simulink model "Trans_2016_DIF_M2_bez_oscilograf"  (R2015a)
settings: Solver=ode23tb  StartTime=0.0  StopTime=4  FixedStep=4e-6  MaxStep=1e-5  RelTol=1e-3  AbsTol=1e-5
values from neighbouring files (symbols this model uses):
  f = 50    [matlab.mat]
  Gm = 6.28318530718e-07    [matlab.mat]
  k = k+1    (= 2)    [SIGMA_trans.m]    (also in matlab.mat = 1e-06)
  LL1 = 0.016    [matlab.mat]
  LL2 = 7.96e-06    [matlab.mat]
  Ln = 0.0060919505207    [matlab.mat]
  R1 = 3.03    [matlab.mat]
  R2 = 0.003    [matlab.mat]
  RL1 = 10    [matlab.mat]
  RL2 = 0.00125    [matlab.mat]
  Rn = 0.63798571162    [matlab.mat]
  S = 0.0216    [matlab.mat]
  w1 = 850    [matlab.mat]
  w2 = 34    [matlab.mat]
undefined symbols (not defined in the file): Lsigma, sigma1, sigma2
libraries: powerlib x77, simulink x1
(part 1 of 2)
settings Model: Creator=Алексей  LastModifiedBy=Aleksey
settings SolverCC: MaxOrder=2  MaxConsecutiveZCs=5.5e6  NumberNewtonIterations=10000  MaxConsecutiveMinStep=1e7  ShapePreserveControl=EnableAll  ZeroCrossAlgorithm=Adaptive  SolverResetMethod=Robust  InsertRTBMode=Always

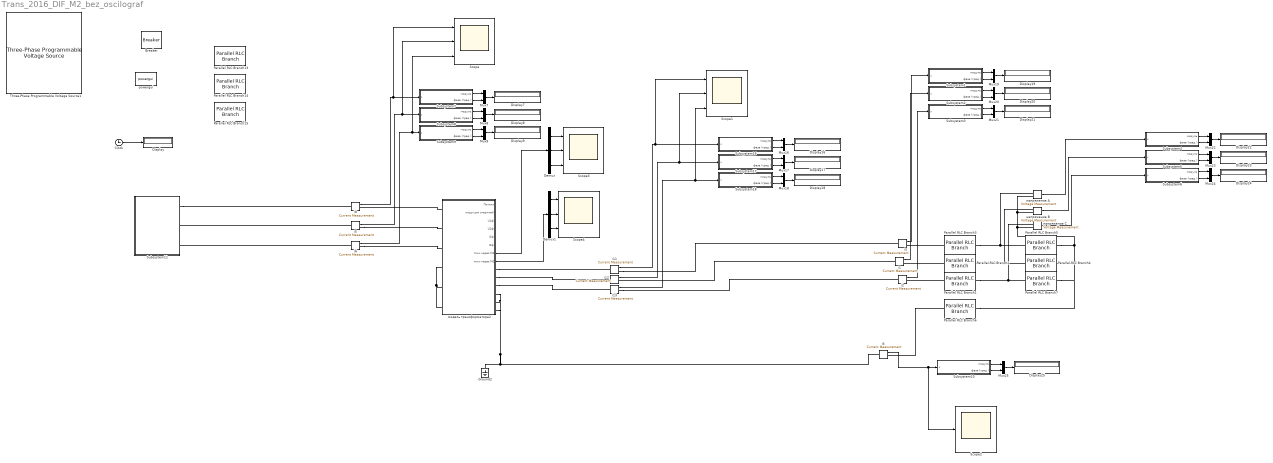
== system Trans_2016_DIF_M2_bez_oscilograf ==
  Breaker : powerlib/Elements/Breaker  InitialState=0  SwitchingTimes="[0.5  2]"  External=off  BreakerResistance=0.01  SnubberResistance=1e6  SnubberCapacitance=inf  Measurements=None  MoreParameters=on  NoBreakLoop=off
  Clock : Clock
  Demux : Demux  Outputs=3
  Demux1 : Demux  Outputs=3
  Display{,7..9,16..25} (14 alike) : Display
      Display16 settings: Decimation=2
      Display17 settings: Decimation=2
      Display18 settings: Decimation=2
      Display19 settings: Decimation=2
      Display20 settings: Decimation=2
      Display21 settings: Decimation=2
      Display22 settings: Decimation=2
      Display23 settings: Decimation=2
      Display24 settings: Decimation=2
      Display25 settings: Decimation=2
      Display7 settings: Decimation=2
      Display8 settings: Decimation=2
      Display9 settings: Decimation=2
  Ground2 : powerlib/Elements/Ground  LConnTagsString=a
  Mux{7..9,16..25} (13 alike) : Mux  Inputs=2
  Parallel RLC Branch{1..3,6} (4 alike) : powerlib/Elements/Parallel RLC Branch  LConnTagsString=a  RConnTagsString=__new0  BranchType=RL  Resistance=RL2  Inductance=LL2  SetiL0=off  InitialCurrent=0  Capacitance=1e-6  Setx0=off  InitialVoltage=0  Measurements=None
  Parallel RLC Branch13 : powerlib/Elements/Parallel RLC Branch  LConnTagsString=a  RConnTagsString=__new0  BranchType=RL  Resistance=RL1  Inductance=LL1  SetiL0=off  InitialCurrent=0  Capacitance=1e-6  Setx0=off  InitialVoltage=0  Measurements=None
  Parallel RLC Branch14 : powerlib/Elements/Parallel RLC Branch  LConnTagsString=a  RConnTagsString=__new0  BranchType=RL  Resistance=RL1  Inductance=LL1  SetiL0=off  InitialCurrent=0  Capacitance=1e-6  Setx0=off  InitialVoltage=0  Measurements=None
  Parallel RLC Branch15 : powerlib/Elements/Parallel RLC Branch  LConnTagsString=a  RConnTagsString=__new0  BranchType=RL  Resistance=RL1  Inductance=LL1  SetiL0=off  InitialCurrent=0  Capacitance=1e-6  Setx0=off  InitialVoltage=0  Measurements=None
  Parallel RLC Branch4 : powerlib/Elements/Parallel RLC Branch  LConnTagsString=a  RConnTagsString=__new0  BranchType=RL  Resistance=Rn  Inductance=Ln  SetiL0=off  InitialCurrent=0  Capacitance=1e-6  Setx0=off  InitialVoltage=0  Measurements=None
  Parallel RLC Branch5 : powerlib/Elements/Parallel RLC Branch  LConnTagsString=a  RConnTagsString=__new0  BranchType=RL  Resistance=Rn  Inductance=Ln  SetiL0=off  InitialCurrent=0  Capacitance=1e-6  Setx0=off  InitialVoltage=0  Measurements=None
  Parallel RLC Branch7 : powerlib/Elements/Parallel RLC Branch  LConnTagsString=a  RConnTagsString=__new0  BranchType=RL  Resistance=Rn  Inductance=Ln  SetiL0=off  InitialCurrent=0  Capacitance=1e-6  Setx0=off  InitialVoltage=0  Measurements=None
  Scope{,1,3..4} (4 alike) : Scope  NumInputPorts=3
      Scope settings: YMin=-19.75~-3.5~15  YMax=-16~5~19.25  MaxDataPoints=20
      Scope1 settings: YMin=-550~-550~-550  YMax=550~550~550  MaxDataPoints=20
      Scope3 settings: YMin=-4~-1~-7.5e-126  YMax=-2.4~1~1.25e-125  SaveName=ScopeData3  MaxDataPoints=20
      Scope4 settings: YMin=2.5e-11~-5.25e-10~1.35e-10  YMax=4e-10~-2.25e-10~2.15e-10  SaveName=ScopeData4  MaxDataPoints=20
  Scope2 : Scope
      settings: YMin=-1  YMax=0.4  SaveName=ScopeData2  MaxDataPoints=20
  Subsystem1 : Subsystem  mask{f=f}
      mask prompts: f "частота"
  Subsystem10 : Subsystem  mask{f=f}
      mask prompts: f "частота"
  Subsystem11 : Subsystem  mask{U=10000, Usek=10000*10/2, f=50}
      mask prompts: U "Линейное U"; Usek "на сколько вырастет напряжение за с"; f "частота"
      mask DialogControl ParameterGroupVar Prompt: Параметры
  Subsystem16 : Subsystem  mask{f=f}
      mask prompts: f "частота"
  Subsystem17 : Subsystem  mask{f=f}
      mask prompts: f "частота"
  Subsystem18 : Subsystem  mask{f=f}
      mask prompts: f "частота"
  Subsystem2 : Subsystem  mask{f=f}
      mask prompts: f "частота"
  Subsystem3 : Subsystem  mask{f=f}
      mask prompts: f "частота"
  Subsystem4 : Subsystem  mask{f=f}
      mask prompts: f "частота"
  Subsystem5 : Subsystem  mask{f=f}
      mask prompts: f "частота"
  Subsystem6 : Subsystem  mask{f=f}
      mask prompts: f "частота"
  Subsystem7 : Subsystem  mask{f=f}
      mask prompts: f "частота"
  Subsystem8 : Subsystem  mask{f=f}
      mask prompts: f "частота"
  Subsystem9 : Subsystem  mask{f=f}
      mask prompts: f "частота"
  Three-Phase Programmable Voltage Source1 : powerlib/Electrical Sources/Three-Phase Programmable Voltage Source  PositiveSequence="[0.01  50 50]"  VariationEntity=Amplitude  VariationType=Ramp  VariationTypeAlt=Step  VariationStep=0.5  VariationRate=10000/sqrt(3)*100*1.225/0.2  VariationMagnitude=0.3  VariationFrequency=2  VariationTiming=[0 0.2]  VariationPhaseA=off  Amplitudes=[1 0.8 1.2 1.0]  TimeValues=[0 0.1 0.15 0.2]  HarmonicGeneration=off  HarmonicA=[3 0.2 -25 0]  HarmonicB=[2 0.15 35 2]  Timing="[0.05  3]"  BusType=swing  Pref=0  Qref=0  Qmin=-inf  Qmax=inf
  i{1..6,8,11..13} (10 alike) : powerlib/Measurements/Current Measurement  PhasorSimulation=off  OutputType=Complex  PSBequivalent=0
  powergui : powerlib/powergui  Priority=1  SimulationMode=Continuous  SolverType=Tustin/Backward Euler (TBE)  SampleTime=50e-6  frequency=60  SPID=off  DisableSnubberDevices=off  DisableRonSwitches=off  DisableVfSwitches=off  SwTol=0  DisplayEquations=off  Interpol=off  methode=off  Ts=100  FunctionMessages=off  echomessages=off  HookPort=off  EnableUseOfTLC=off  x0status=blocks  frequencyindice=0  Pbase=100e6  ErrMax=1e-4  Iterations=50  UnitsV=kV  UnitsW=MW  buscounter=0  RestoreLinks=warning  ResistiveCurrentMeasurement=off  Frange=[0:2:500]  Ylog=off  Xlog=on  ShowGrid=off  save=off  variable=ZData  structure=0  ZoomFFT=off  StartTime=0.0  cycles=1  DisplayStyle=1  fundamental=60  FreqAxis=off  MaxFrequency=1000  frequencyindicesteady=1  RmsSteady=1  display=off
  модель трансформатора2 : Subsystem  mask{S=S, w1=w1, w2=w2, R1=R1, R2=R2, Lsigmavx=Lsigma, Sigma1=sigma1, Sigma2=sigma2, Gm=Gm, w1_do=[850 850 850], w2_do=[34 34 34], w1_posle=[850-21 850-21 850-21], w2_posle=[34 34 34], tRPN=0.3, tstup=0.1}
      mask prompts: S "Площадь сердечника"; w1 "Номинальное количество витков в первичной обмотке"; w2 "Номинальное количество витков в вторичной обмотке"; R1 "Активное сопротивление проводов первичной обмотки"; R2 "Сопротивление проводов вторичной обмотки"; Lsigmavx "индуктивность расеивания обмоток (квадратная матрица)"; Sigma1 "Участок сигма 1"; Sigma2 "Участок сигма 2"; Gm "Проводимость по воздуху"; w1_do "Матрица витков в первичке до срабатывания (1x3)"; w2_do "Матрица витков во вторичке до срабатывания (1x3)"; w1_posle "Матрица витков в первичке после срабатывания (1x3)"; w2_posle "Матрица витков во вторичке после срабатывания (1x3)"; tRPN "Время срабаотывания РПН"; tstup "Время шага ступени"
      mask DialogControl Container3 Prompt: Кривая намагничивания (матрицы должы быть одной размерности)
  напряжение А : powerlib/Measurements/Voltage Measurement  PhasorSimulation=off  OutputType=Complex  PSBequivalent=0
  напряжение В : powerlib/Measurements/Voltage Measurement  PhasorSimulation=off  OutputType=Complex  PSBequivalent=0
  напряжение С : powerlib/Measurements/Voltage Measurement  PhasorSimulation=off  OutputType=Complex  PSBequivalent=0
  wires:
  Clock/1 -> Display/1
  i3/1 -> Subsystem1/1(х)
  i1/1 -> Subsystem2/1(х)
  i2/1 -> Subsystem3/1(х)
  напряжение С/1 -> Subsystem6/1(х)
  напряжение В/1 -> Subsystem5/1(х)
  напряжение А/1 -> Subsystem4/1(х)
  i13/1 -> Scope1/3, Subsystem18/1(х)
  i11/1 -> Scope1/1, Subsystem16/1(х)
  Subsystem7/1(модуль) -> Mux7/1
  Subsystem7/2(фаза (град.)) -> Mux7/2
  Mux7/1 -> Display7/1
  Subsystem8/1(модуль) -> Mux8/1
  Subsystem8/2(фаза (град.)) -> Mux8/2
  Mux8/1 -> Display8/1
  Subsystem9/1(модуль) -> Mux9/1
  Subsystem9/2(фаза (град.)) -> Mux9/2
  Mux9/1 -> Display9/1
  Subsystem16/1(модуль) -> Mux16/1
  Subsystem16/2(фаза (град.)) -> Mux16/2
  Mux16/1 -> Display16/1
  Subsystem17/1(модуль) -> Mux17/1
  Subsystem17/2(фаза (град.)) -> Mux17/2
  Mux17/1 -> Display17/1
  Subsystem18/1(модуль) -> Mux18/1
  Subsystem18/2(фаза (град.)) -> Mux18/2
  Mux18/1 -> Display18/1
  Subsystem1/1(модуль) -> Mux19/1
  Subsystem1/2(фаза (град.)) -> Mux19/2
  Mux19/1 -> Display19/1
  Subsystem2/1(модуль) -> Mux20/1
  Subsystem2/2(фаза (град.)) -> Mux20/2
  Mux20/1 -> Display20/1
  Subsystem3/1(модуль) -> Mux21/1
  Subsystem3/2(фаза (град.)) -> Mux21/2
  Mux21/1 -> Display21/1
  Subsystem4/1(модуль) -> Mux22/1
  Subsystem4/2(фаза (град.)) -> Mux22/2
  Mux22/1 -> Display22/1
  Subsystem5/1(модуль) -> Mux23/1
  Subsystem5/2(фаза (град.)) -> Mux23/2
  Mux23/1 -> Display23/1
  Subsystem6/1(модуль) -> Mux24/1
  Subsystem6/2(фаза (град.)) -> Mux24/2
  Mux24/1 -> Display24/1
  Subsystem10/2(фаза (град.)) -> Mux25/2
  Mux25/1 -> Display25/1
  Subsystem10/1(модуль) -> Mux25/1
  i8/1 -> Scope/1, Subsystem7/1(х)
  i5/1 -> Subsystem8/1(х), Scope/2
  i6/1 -> Scope/3, Subsystem9/1(х)
  i12/1 -> Scope1/2, Subsystem17/1(х)
  i4/1 -> Scope2/1, Subsystem10/1(х)
  Demux/1 -> Scope3/1
  Demux/2 -> Scope3/2
  Demux/3 -> Scope3/3
  модель трансформатора2/7(токи через М1) -> Demux/1
  Demux1/1 -> Scope4/1
  Demux1/2 -> Scope4/2
  Demux1/3 -> Scope4/3
  модель трансформатора2/8(токи через М2) -> Demux1/1
  connections:
  модель трансформатора2/RConn3 -- i13/LConn1
  модель трансформатора2/RConn1 -- i11/LConn1
  модель трансформатора2/RConn2 -- i12/LConn1
  модель трансформатора2/RConn6 -- модель трансформатора2/RConn4 -- модель трансформатора2/RConn5 -- i4/LConn1 -- Ground2/LConn1
  Parallel RLC Branch3/RConn1 -- Parallel RLC Branch5/LConn1 -- напряжение А/LConn1
  Parallel RLC Branch2/RConn1 -- Parallel RLC Branch4/LConn1 -- напряжение В/LConn1
  Parallel RLC Branch1/RConn1 -- Parallel RLC Branch7/LConn1 -- напряжение С/LConn1
  Parallel RLC Branch3/LConn1 -- i3/RConn1
  Parallel RLC Branch2/LConn1 -- i1/RConn1
  Parallel RLC Branch1/LConn1 -- i2/RConn1
  i11/RConn1 -- i3/LConn1
  i1/LConn1 -- i12/RConn1
  i13/RConn1 -- i2/LConn1
  Parallel RLC Branch7/RConn1 -- Parallel RLC Branch6/RConn1 -- Parallel RLC Branch4/RConn1 -- Parallel RLC Branch5/RConn1 -- напряжение С/LConn2 -- напряжение А/LConn2 -- напряжение В/LConn2
  Parallel RLC Branch6/LConn1 -- i4/RConn1
  модель трансформатора2/LConn4 -- модель трансформатора2/LConn5 -- модель трансформатора2/LConn6
  модель трансформатора2/LConn1 -- i8/RConn1
  i6/RConn1 -- модель трансформатора2/LConn3
  i5/RConn1 -- модель трансформатора2/LConn2
  Subsystem11/RConn1 -- i8/LConn1
  i5/LConn1 -- Subsystem11/RConn2
  i6/LConn1 -- Subsystem11/RConn3

== system Trans_2016_DIF_M2_bez_oscilograf/Subsystem1 ==
  х : Inport
  Subsystem : Subsystem  mask{f=f}
      mask prompts: f "частота"
      mask DialogControl ParameterGroupVar Prompt: параметры
  Subsystem4 : Subsystem  mask{T=1/f}
      mask prompts: T "период"
  zader : Memory
  модуль : Outport
  фаза (град.) : Outport  Port=2
  wires:
  х/1 -> zader/1
  Subsystem4/1(фаза) -> фаза (град.)/1
  zader/1 -> Subsystem/1(x), Subsystem4/1(х)
  Subsystem/1(deystv) -> модуль/1

== system Trans_2016_DIF_M2_bez_oscilograf/Subsystem10 ==
  х : Inport
  Subsystem : Subsystem  mask{f=f}
      mask prompts: f "частота"
      mask DialogControl ParameterGroupVar Prompt: параметры
  Subsystem4 : Subsystem  mask{T=1/f}
      mask prompts: T "период"
  zader : Memory
  модуль : Outport
  фаза (град.) : Outport  Port=2
  wires:
  х/1 -> zader/1
  Subsystem4/1(фаза) -> фаза (град.)/1
  zader/1 -> Subsystem/1(x), Subsystem4/1(х)
  Subsystem/1(deystv) -> модуль/1

== system Trans_2016_DIF_M2_bez_oscilograf/Subsystem11 ==
  Controlled Voltage Source : powerlib/Electrical Sources/Controlled Voltage Source  Initialize=on  Source_Type=AC  Amplitude=0  Phase=0  Frequency=0  Measurements=None
  Controlled Voltage Source1 : powerlib/Electrical Sources/Controlled Voltage Source  Initialize=on  Source_Type=AC  Amplitude=0  Phase=0  Frequency=0  Measurements=None
  Divide : Product  Inputs=**
  Divide1 : Product  Inputs=**
  Ramp : simulink/Sources/Ramp  slope=Usek  start=0  X0=0
  Saturation : Saturate  UpperLimit=U  LowerLimit=0
  Sine Wave : Sin  Amplitude=1*sqrt(2)  Frequency=f*2*pi  SampleTime=0
  Sine Wave1 : Sin  Amplitude=1*sqrt(2)  Frequency=f*2*pi  Phase=-120/360*2*pi  SampleTime=0
  Conn1 : PMIOPort  Port=1  Side=Right
  Conn2 : PMIOPort  Port=2  Side=Right
  Conn3 : PMIOPort  Port=3  Side=Right
  wires:
  Saturation/1 -> Divide1/1, Divide/2
  Divide1/1 -> Controlled Voltage Source1/1
  Sine Wave/1 -> Divide/1
  Divide/1 -> Controlled Voltage Source/1
  Sine Wave1/1 -> Divide1/2
  Ramp/1 -> Saturation/1
  connections:
  Controlled Voltage Source1/LConn1 -- Conn3/RConn1
  Controlled Voltage Source/RConn1 -- Conn1/RConn1
  Controlled Voltage Source1/RConn1 -- Controlled Voltage Source/LConn1 -- Conn2/RConn1

== system Trans_2016_DIF_M2_bez_oscilograf/Subsystem16 ==
  х : Inport
  Subsystem : Subsystem  mask{f=f}
      mask prompts: f "частота"
      mask DialogControl ParameterGroupVar Prompt: параметры
  Subsystem4 : Subsystem  mask{T=1/f}
      mask prompts: T "период"
  zader : Memory
  модуль : Outport
  фаза (град.) : Outport  Port=2
  wires:
  Subsystem/1(deystv) -> модуль/1
  zader/1 -> Subsystem4/1(х), Subsystem/1(x)
  Subsystem4/1(фаза) -> фаза (град.)/1
  х/1 -> zader/1

== system Trans_2016_DIF_M2_bez_oscilograf/Subsystem17 ==
  х : Inport
  Subsystem : Subsystem  mask{f=f}
      mask prompts: f "частота"
      mask DialogControl ParameterGroupVar Prompt: параметры
  Subsystem4 : Subsystem  mask{T=1/f}
      mask prompts: T "период"
  zader : Memory
  модуль : Outport
  фаза (град.) : Outport  Port=2
  wires:
  х/1 -> zader/1
  Subsystem4/1(фаза) -> фаза (град.)/1
  zader/1 -> Subsystem/1(x), Subsystem4/1(х)
  Subsystem/1(deystv) -> модуль/1

== system Trans_2016_DIF_M2_bez_oscilograf/Subsystem18 ==
  х : Inport
  Subsystem : Subsystem  mask{f=f}
      mask prompts: f "частота"
      mask DialogControl ParameterGroupVar Prompt: параметры
  Subsystem4 : Subsystem  mask{T=1/f}
      mask prompts: T "период"
  zader : Memory
  модуль : Outport
  фаза (град.) : Outport  Port=2
  wires:
  Subsystem/1(deystv) -> модуль/1
  zader/1 -> Subsystem4/1(х), Subsystem/1(x)
  Subsystem4/1(фаза) -> фаза (град.)/1
  х/1 -> zader/1

== system Trans_2016_DIF_M2_bez_oscilograf/Subsystem2 ==
  х : Inport
  Subsystem : Subsystem  mask{f=f}
      mask prompts: f "частота"
      mask DialogControl ParameterGroupVar Prompt: параметры
  Subsystem4 : Subsystem  mask{T=1/f}
      mask prompts: T "период"
  zader : Memory
  модуль : Outport
  фаза (град.) : Outport  Port=2
  wires:
  Subsystem/1(deystv) -> модуль/1
  zader/1 -> Subsystem4/1(х), Subsystem/1(x)
  Subsystem4/1(фаза) -> фаза (град.)/1
  х/1 -> zader/1

== system Trans_2016_DIF_M2_bez_oscilograf/Subsystem3 ==
  х : Inport
  Subsystem : Subsystem  mask{f=f}
      mask prompts: f "частота"
      mask DialogControl ParameterGroupVar Prompt: параметры
  Subsystem4 : Subsystem  mask{T=1/f}
      mask prompts: T "период"
  zader : Memory
  модуль : Outport
  фаза (град.) : Outport  Port=2
  wires:
  х/1 -> zader/1
  Subsystem4/1(фаза) -> фаза (град.)/1
  zader/1 -> Subsystem/1(x), Subsystem4/1(х)
  Subsystem/1(deystv) -> модуль/1

== system Trans_2016_DIF_M2_bez_oscilograf/Subsystem4 ==
  х : Inport
  Subsystem : Subsystem  mask{f=f}
      mask prompts: f "частота"
      mask DialogControl ParameterGroupVar Prompt: параметры
  Subsystem4 : Subsystem  mask{T=1/f}
      mask prompts: T "период"
  zader : Memory
  модуль : Outport
  фаза (град.) : Outport  Port=2
  wires:
  Subsystem/1(deystv) -> модуль/1
  zader/1 -> Subsystem4/1(х), Subsystem/1(x)
  Subsystem4/1(фаза) -> фаза (град.)/1
  х/1 -> zader/1

== system Trans_2016_DIF_M2_bez_oscilograf/Subsystem5 ==
  х : Inport
  Subsystem : Subsystem  mask{f=f}
      mask prompts: f "частота"
      mask DialogControl ParameterGroupVar Prompt: параметры
  Subsystem4 : Subsystem  mask{T=1/f}
      mask prompts: T "период"
  zader : Memory
  модуль : Outport
  фаза (град.) : Outport  Port=2
  wires:
  х/1 -> zader/1
  Subsystem4/1(фаза) -> фаза (град.)/1
  zader/1 -> Subsystem/1(x), Subsystem4/1(х)
  Subsystem/1(deystv) -> модуль/1

== system Trans_2016_DIF_M2_bez_oscilograf/Subsystem6 ==
  х : Inport
  Subsystem : Subsystem  mask{f=f}
      mask prompts: f "частота"
      mask DialogControl ParameterGroupVar Prompt: параметры
  Subsystem4 : Subsystem  mask{T=1/f}
      mask prompts: T "период"
  zader : Memory
  модуль : Outport
  фаза (град.) : Outport  Port=2
  wires:
  Subsystem/1(deystv) -> модуль/1
  zader/1 -> Subsystem4/1(х), Subsystem/1(x)
  Subsystem4/1(фаза) -> фаза (град.)/1
  х/1 -> zader/1

== system Trans_2016_DIF_M2_bez_oscilograf/Subsystem7 ==
  х : Inport
  Subsystem : Subsystem  mask{f=f}
      mask prompts: f "частота"
      mask DialogControl ParameterGroupVar Prompt: параметры
  Subsystem4 : Subsystem  mask{T=1/f}
      mask prompts: T "период"
  zader : Memory
  модуль : Outport
  фаза (град.) : Outport  Port=2
  wires:
  х/1 -> zader/1
  Subsystem4/1(фаза) -> фаза (град.)/1
  zader/1 -> Subsystem/1(x), Subsystem4/1(х)
  Subsystem/1(deystv) -> модуль/1

== system Trans_2016_DIF_M2_bez_oscilograf/Subsystem8 ==
  х : Inport
  Subsystem : Subsystem  mask{f=f}
      mask prompts: f "частота"
      mask DialogControl ParameterGroupVar Prompt: параметры
  Subsystem4 : Subsystem  mask{T=1/f}
      mask prompts: T "период"
  zader : Memory
  модуль : Outport
  фаза (град.) : Outport  Port=2
  wires:
  Subsystem/1(deystv) -> модуль/1
  zader/1 -> Subsystem4/1(х), Subsystem/1(x)
  Subsystem4/1(фаза) -> фаза (град.)/1
  х/1 -> zader/1

== system Trans_2016_DIF_M2_bez_oscilograf/Subsystem9 ==
  х : Inport
  Subsystem : Subsystem  mask{f=f}
      mask prompts: f "частота"
      mask DialogControl ParameterGroupVar Prompt: параметры
  Subsystem4 : Subsystem  mask{T=1/f}
      mask prompts: T "период"
  zader : Memory
  модуль : Outport
  фаза (град.) : Outport  Port=2
  wires:
  х/1 -> zader/1
  Subsystem4/1(фаза) -> фаза (град.)/1
  zader/1 -> Subsystem/1(x), Subsystem4/1(х)
  Subsystem/1(deystv) -> модуль/1

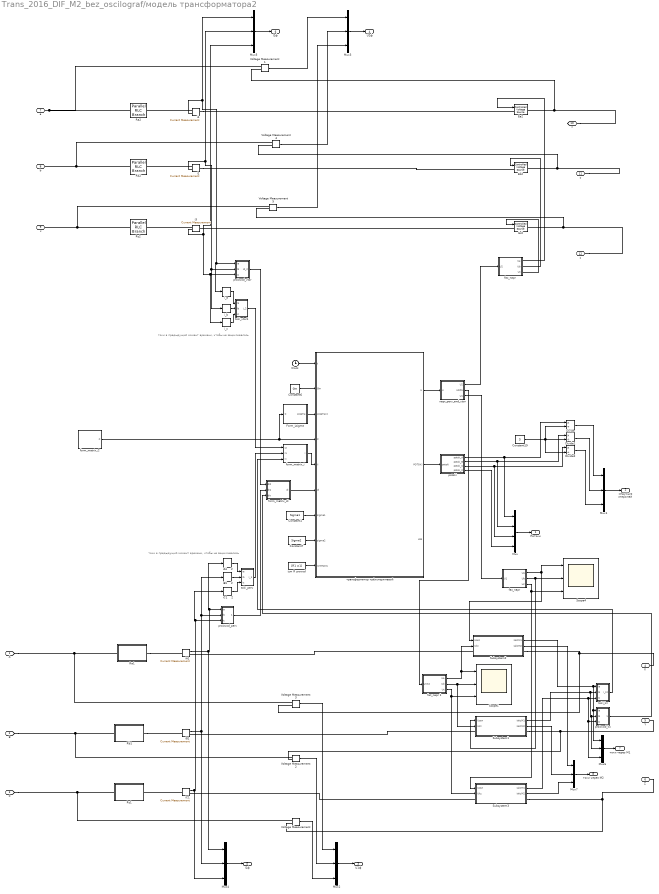
== system Trans_2016_DIF_M2_bez_oscilograf/модель трансформатора2 ==
  note: токи в предыдущий момент времени, чтобы не зацикливалось
  note: токи в предыдущий момент времени, чтобы не зацикливалось
  Clock : Clock
  Constant1 : Constant  Value=Sigma1
  Constant19 : Constant  Value=S
  Constant6 : Constant  Value=Gm
  Constant7 : Constant  Value=Sigma2
  Divide : Product  Inputs=*/
  Divide1 : Product  Inputs=*/
  Divide2 : Product  Inputs=*/
  Ea2 : powerlib/Electrical Sources/Controlled Voltage Source  Initialize=on  Source_Type=AC  Amplitude=0  Phase=0  Frequency=0  Measurements=None
  Eb2 : powerlib/Electrical Sources/Controlled Voltage Source  Initialize=on  Source_Type=AC  Amplitude=0  Phase=0  Frequency=0  Measurements=None
  Ec2 : powerlib/Electrical Sources/Controlled Voltage Source  Initialize=on  Source_Type=AC  Amplitude=0  Phase=0  Frequency=0  Measurements=None
  Form_Lsigma : Subsystem
  Mux : Mux
  Mux{1..7} (7 alike) : Mux  Inputs=3
  Ra1 : Subsystem  mask{t=1e-4, r=R1}
      mask prompts: t "время включения"; r "сопротивление обмотки"
  Ra2 : powerlib/Elements/Parallel RLC Branch  LConnTagsString=a  RConnTagsString=__new0  BranchType=R  Resistance=R2  Inductance=1e-3  SetiL0=off  InitialCurrent=0  Capacitance=1e-6  Setx0=off  InitialVoltage=0  Measurements=None
  Rb1 : Subsystem  mask{t=1e-4, r=R1}
      mask prompts: t "время включения"; r "сопротивление обмотки"
  Rb2 : powerlib/Elements/Parallel RLC Branch  LConnTagsString=a  RConnTagsString=__new0  BranchType=R  Resistance=R2  Inductance=1e-3  SetiL0=off  InitialCurrent=0  Capacitance=1e-6  Setx0=off  InitialVoltage=0  Measurements=None
  Rc1 : Subsystem  mask{t=1e-4, r=R1}
      mask prompts: t "время включения"; r "сопротивление обмотки"
  Rс2 : powerlib/Elements/Parallel RLC Branch  LConnTagsString=a  RConnTagsString=__new0  BranchType=R  Resistance=R2  Inductance=1e-3  SetiL0=off  InitialCurrent=0  Capacitance=1e-6  Setx0=off  InitialVoltage=0  Measurements=None
  Scope1 : Scope  NumInputPorts=3
      settings: YMin=97~-1.8e+08~1.75e+08  YMax=113~-5e+07~6e+08  SaveName=ScopeData6  MaxDataPoints=20
  Scope4 : Scope  NumInputPorts=3
      settings: YMin=500~-5000~-8250  YMax=8500~7000~-3250  SaveName=ScopeData5  MaxDataPoints=20
  Subsystem1 : Subsystem  mask{tRPN=tRPN, tstup=tstup, Rrpn=4}
      mask prompts: tRPN "время срабатывания РПН (с)"; tstup "шаг ступени РПН(с)"; Rrpn "сопротивление резисторов в цепи РПН (Ом)"
  Subsystem2 : Subsystem  mask{tRPN=tRPN, tstup=tstup, Rrpn=4}
      mask prompts: tRPN "время срабатывания РПН (с)"; tstup "шаг ступени РПН(с)"; Rrpn "сопротивление резисторов в цепи РПН (Ом)"
  Subsystem3 : Subsystem  mask{tRPN=tRPN, tstup=tstup, Rrpn=4}
      mask prompts: tRPN "время срабатывания РПН (с)"; tstup "шаг ступени РПН(с)"; Rrpn "сопротивление резисторов в цепи РПН (Ом)"
  Voltage Measurement{,1..5} (6 alike) : powerlib/Measurements/Voltage Measurement  PhasorSimulation=off  OutputType=Complex  PSBequivalent=0
  faz_napr : Subsystem
  "faz_napr " : Subsystem
  faz_napr 1 : Subsystem
  "form_matrix_C " : Subsystem  mask{tRPN=tRPN, tstup=tstup}
      mask prompts: tRPN "время срабатывания РПН"; tstup "время шага ступени РПН (с)"
  form_matrix_di : Subsystem
  form_matrix_i : Subsystem
  i1 : powerlib/Measurements/Current Measurement  PhasorSimulation=off  OutputType=Complex  PSBequivalent=0
  i3 : powerlib/Measurements/Current Measurement  PhasorSimulation=off  OutputType=Complex  PSBequivalent=0
  i4 : powerlib/Measurements/Current Measurement  PhasorSimulation=off  OutputType=Complex  PSBequivalent=0
  iA1 : powerlib/Measurements/Current Measurement  PhasorSimulation=off  OutputType=Complex  PSBequivalent=0
  iA1    2 : Memory
  iB1 : powerlib/Measurements/Current Measurement  PhasorSimulation=off  OutputType=Complex  PSBequivalent=0
  iB1    2 : Memory
  iC1 : powerlib/Measurements/Current Measurement  PhasorSimulation=off  OutputType=Complex  PSBequivalent=0
      link override source: GotoTag=T55_24746_511570940550896
  iC1    2 : Memory
  i_a : Memory
  i_b : Memory
  i_c : Memory
  izm R provod : Constant  Value=[R1 w1]
  napr_perv_and_vtor : Subsystem
  potoki : Subsystem
  proizvod_kz : Subsystem
  proizvod_perv : Subsystem
  proizvod_vtor : Subsystem
  toki_kz : Subsystem
  toki_perv : Subsystem
  toki_vtor1 : Subsystem
  трансформатор трёхстержневой : MATLAB Function  TreatAsAtomicUnit=on
  А : PMIOPort  Port=1  Side=Left
  В : PMIOPort  Port=2  Side=Left
  С : PMIOPort  Port=3  Side=Left
  Х : PMIOPort  Port=4  Side=Left
  Y : PMIOPort  Port=5  Side=Left
  Z : PMIOPort  Port=6  Side=Left
  a : PMIOPort  Port=7  Side=Right
  b : PMIOPort  Port=8  Side=Right
  c : PMIOPort  Port=9  Side=Right
  x : PMIOPort  Port=10  Side=Right
  y : PMIOPort  Port=11  Side=Right
  z : PMIOPort  Port=12  Side=Right
  Потоки : Outport
  индукция стержней : Outport  Port=2
  U1ф : Outport  Port=3
  U2ф : Outport  Port=4
  I1ф : Outport  Port=5
  I2ф : Outport  Port=6
  токи через М1 : Outport  Port=7
  токи через М2 : Outport  Port=8
  wires:
  iC1/1 -> Mux4/3, proizvod_perv/3(ic), iC1    2/1
  iB1/1 -> Mux4/2, proizvod_perv/2(ib), iB1    2/1
  iA1/1 -> Mux4/1, proizvod_perv/1(ia), iA1    2/1
  i4/1 -> proizvod_vtor/1(ia), i_a/1, Mux5/1
  i1/1 -> i_b/1, proizvod_vtor/2(ib), Mux5/2
  i3/1 -> Mux5/3, i_c/1, proizvod_vtor/3(ic)
  "form_matrix_C "/1(C) -> трансформатор трёхстержневой/4(C), Form_Lsigma/1(C)
  Mux/1 -> Потоки/1
  Mux5/1 -> I2ф/1
  Mux4/1 -> I1ф/1
  Voltage Measurement5/1 -> Mux3/3
  Voltage Measurement4/1 -> Mux3/2
  Voltage Measurement1/1 -> Mux3/1
  Mux3/1 -> U2ф/1
  Voltage Measurement/1 -> Mux2/3
  Voltage Measurement2/1 -> Mux2/2
  Voltage Measurement3/1 -> Mux2/1
  Mux2/1 -> U1ф/1
  Divide2/1 -> Mux1/3
  Mux1/1 -> индукция стержней/1
  Divide1/1 -> Mux1/2
  Constant19/1 -> Divide/2, Divide1/2, Divide2/2
  Divide/1 -> Mux1/1
  toki_vtor1/1(i_2) -> form_matrix_i/1(i2)
  toki_perv/1(i_1) -> form_matrix_i/2("i1 ")
  iB1    2/1 -> toki_perv/2(ib)
  iA1    2/1 -> toki_perv/1(ia)
  iC1    2/1 -> toki_perv/3(ic)
  i_b/1 -> toki_vtor1/2(ib)
  i_c/1 -> toki_vtor1/3(ic)
  i_a/1 -> toki_vtor1/1(ia)
  proizvod_vtor/1(di_2) -> form_matrix_di/1(di2)
  proizvod_perv/1(di_1) -> form_matrix_di/2("di1 ")
  form_matrix_i/1(i) -> трансформатор трёхстержневой/5(ii)
  form_matrix_di/1(di) -> трансформатор трёхстержневой/6(di)
  Constant7/1 -> трансформатор трёхстержневой/8(sigma2)
  Constant1/1 -> трансформатор трёхстержневой/7(sigma1)
  Constant6/1 -> трансформатор трёхстержневой/2(Gm)
  Clock/1 -> трансформатор трёхстержневой/1(t)
  трансформатор трёхстержневой/1(U) -> napr_perv_and_vtor/1(U)
  "faz_napr "/2(Ub) -> Subsystem1/1(Uosn), Scope4/2
  "faz_napr "/3(Uc) -> Subsystem3/1(Uosn), Scope4/3
  napr_perv_and_vtor/3(U1) -> "faz_napr "/1("U1 ")
  faz_napr/1(Ua) -> Ea2/1
  faz_napr/2(Ub) -> Eb2/1
  faz_napr/3(Uc) -> Ec2/1
  napr_perv_and_vtor/1(U2) -> faz_napr/1("U2 ")
  трансформатор трёхстержневой/2(POTOKI) -> potoki/1("potoki ")
  potoki/1(potok_A) -> Mux/1, Divide/1
  potoki/2(potok_B) -> Mux/2, Divide1/1
  potoki/3(potok_C) -> Mux/3, Divide2/1
  potoki/4(potok_0) -> Mux/4
  Form_Lsigma/1(Lsigma) -> трансформатор трёхстержневой/3(Lsigmavx)
  izm R provod/1 -> трансформатор трёхстержневой/9(izmRprov)
  "faz_napr "/1(Ua) -> Subsystem2/1(Uosn), Scope4/1
  napr_perv_and_vtor/2(URPN) -> faz_napr 1/1("UvKZ ")
  faz_napr 1/1(Ua) -> Subsystem2/2(Ukz), Scope1/1
  faz_napr 1/2(Ub) -> Subsystem1/2(Ukz), Scope1/2
  faz_napr 1/3(Uc) -> Subsystem3/2(Ukz), Scope1/3
  Subsystem2/1(iakzM1) -> Mux6/1, proizvod_kz/1(ia), toki_kz/1(ia)
  Subsystem3/1(iakzM1) -> Mux6/3, proizvod_kz/3(ic), toki_kz/3(ic)
  toki_kz/1(i_kz) -> form_matrix_i/3(iv)
  proizvod_kz/1(di_kz) -> form_matrix_di/3(div)
  Mux6/1 -> токи через М1/1
  Subsystem1/1(iakzM1) -> Mux6/2, proizvod_kz/2(ib), toki_kz/2(ib)
  Mux7/1 -> токи через М2/1
  Subsystem2/2(iakzM2) -> Mux7/1
  Subsystem1/2(iakzM2) -> Mux7/2
  Subsystem3/2(iakzM2) -> Mux7/3
  connections:
  Voltage Measurement4/LConn2 -- y/RConn1 -- Eb2/RConn1
  x/RConn1 -- Voltage Measurement1/LConn2 -- Ea2/RConn1
  Voltage Measurement2/LConn2 -- Subsystem1/RConn1 -- Y/RConn1
  i4/LConn1 -- Ea2/LConn1
  i1/LConn1 -- Eb2/LConn1
  Subsystem3/LConn1 -- iC1/RConn1
  Subsystem1/LConn1 -- iB1/RConn1
  i3/LConn1 -- Ec2/LConn1
  z/RConn1 -- Voltage Measurement5/LConn2 -- Ec2/RConn1
  Voltage Measurement5/LConn1 -- Rс2/LConn1 -- c/RConn1
  Voltage Measurement4/LConn1 -- Rb2/LConn1 -- b/RConn1
  a/RConn1 -- Ra2/LConn1 -- Voltage Measurement1/LConn1
  iC1/LConn1 -- Rc1/RConn1
  Rb1/RConn1 -- iB1/LConn1
  Ra1/RConn1 -- iA1/LConn1
  i1/RConn1 -- Rb2/RConn1
  i3/RConn1 -- Rс2/RConn1
  i4/RConn1 -- Ra2/RConn1
  А/RConn1 -- Ra1/LConn1 -- Voltage Measurement3/LConn1
  Voltage Measurement2/LConn1 -- Rb1/LConn1 -- В/RConn1
  С/RConn1 -- Voltage Measurement/LConn1 -- Rc1/LConn1
  Z/RConn1 -- Subsystem3/RConn1 -- Voltage Measurement/LConn2
  Voltage Measurement3/LConn2 -- Subsystem2/RConn1 -- Х/RConn1
  Subsystem2/LConn1 -- iA1/RConn1

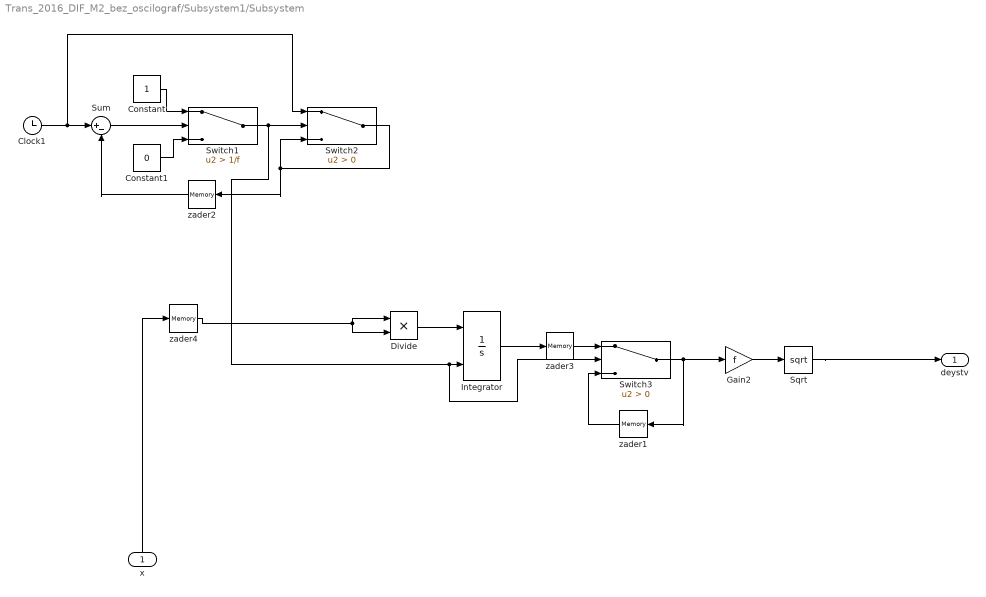
== system Trans_2016_DIF_M2_bez_oscilograf/Subsystem1/Subsystem ==
  x : Inport
  Clock1 : Clock
  Constant : Constant
  Constant1 : Constant  Value=0
  Divide : Product  Inputs=**
  Gain2 : Gain  Gain=f
  Integrator : Integrator  ExternalReset=level
  Sqrt : Sqrt  SaturateOnIntegerOverflow=on
  Sum : Sum  Inputs=|+-
  Switch1 : Switch  Criteria=u2 > Threshold  Threshold=1/f
  Switch2 : Switch  Criteria=u2 > Threshold
  Switch3 : Switch  Criteria=u2 > Threshold
  zader{1..4} (4 alike) : Memory
  deystv : Outport
  wires:
  Integrator/1 -> zader3/1
  Clock1/1 -> Switch2/1, Sum/1
  Switch2/1 -> zader2/1, Switch2/3
  x/1 -> zader4/1
  Constant/1 -> Switch1/1
  Switch1/1 -> Switch3/2, Integrator/2, Switch2/2
  Constant1/1 -> Switch1/3
  Sum/1 -> Switch1/2
  Divide/1 -> Integrator/1
  Switch3/1 -> Gain2/1, zader1/1
  Sqrt/1 -> deystv/1
  Gain2/1 -> Sqrt/1
  zader2/1 -> Sum/2
  zader1/1 -> Switch3/3
  zader3/1 -> Switch3/1
  zader4/1 -> Divide/1, Divide/2

== system Trans_2016_DIF_M2_bez_oscilograf/Subsystem1/Subsystem4 ==
  х : Inport
  Clock1 : Clock
  Constant : Constant  Value=T
  MATLAB Function : MATLAB Function  TreatAsAtomicUnit=on
  zader : Memory
  zader1 : Memory
  фаза : Outport
  wires:
  MATLAB Function/1(y) -> фаза/1, zader1/1
  zader/1 -> MATLAB Function/4(x_pred)
  Clock1/1 -> MATLAB Function/1(t)
  х/1 -> zader/1, MATLAB Function/3(x)
  Constant/1 -> MATLAB Function/2(T_period)
  zader1/1 -> MATLAB Function/5(y_pred)

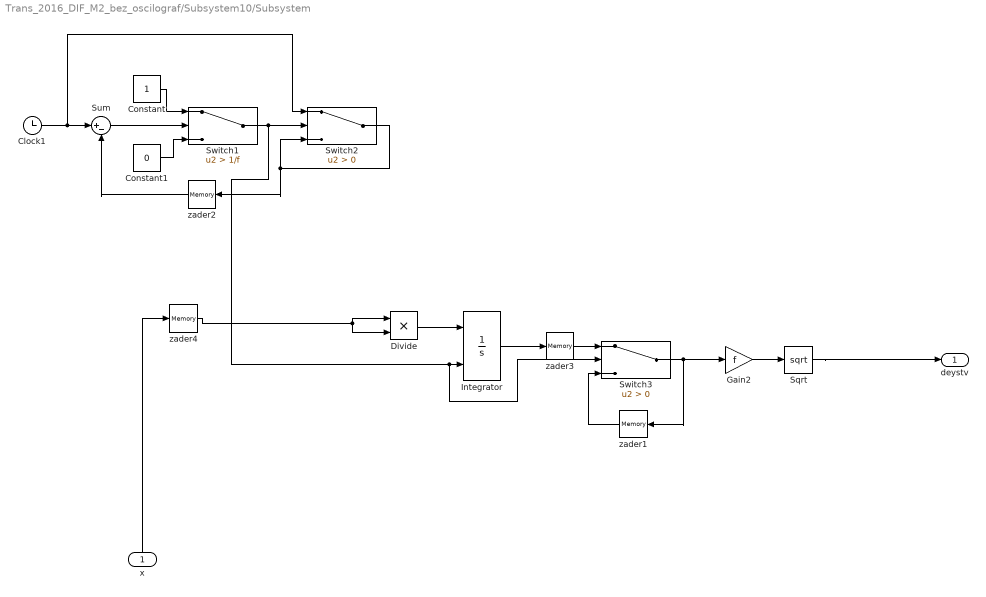
== system Trans_2016_DIF_M2_bez_oscilograf/Subsystem10/Subsystem ==
  x : Inport
  Clock1 : Clock
  Constant : Constant
  Constant1 : Constant  Value=0
  Divide : Product  Inputs=**
  Gain2 : Gain  Gain=f
  Integrator : Integrator  ExternalReset=level
  Sqrt : Sqrt  SaturateOnIntegerOverflow=on
  Sum : Sum  Inputs=|+-
  Switch1 : Switch  Criteria=u2 > Threshold  Threshold=1/f
  Switch2 : Switch  Criteria=u2 > Threshold
  Switch3 : Switch  Criteria=u2 > Threshold
  zader{1..4} (4 alike) : Memory
  deystv : Outport
  wires:
  Integrator/1 -> zader3/1
  Clock1/1 -> Switch2/1, Sum/1
  Switch2/1 -> zader2/1, Switch2/3
  x/1 -> zader4/1
  Constant/1 -> Switch1/1
  Switch1/1 -> Switch3/2, Integrator/2, Switch2/2
  Constant1/1 -> Switch1/3
  Sum/1 -> Switch1/2
  Divide/1 -> Integrator/1
  Switch3/1 -> Gain2/1, zader1/1
  Sqrt/1 -> deystv/1
  Gain2/1 -> Sqrt/1
  zader2/1 -> Sum/2
  zader1/1 -> Switch3/3
  zader3/1 -> Switch3/1
  zader4/1 -> Divide/1, Divide/2

== system Trans_2016_DIF_M2_bez_oscilograf/Subsystem10/Subsystem4 ==
  х : Inport
  Clock1 : Clock
  Constant : Constant  Value=T
  MATLAB Function : MATLAB Function  TreatAsAtomicUnit=on
  zader : Memory
  zader1 : Memory
  фаза : Outport
  wires:
  MATLAB Function/1(y) -> фаза/1, zader1/1
  zader/1 -> MATLAB Function/4(x_pred)
  Clock1/1 -> MATLAB Function/1(t)
  х/1 -> zader/1, MATLAB Function/3(x)
  Constant/1 -> MATLAB Function/2(T_period)
  zader1/1 -> MATLAB Function/5(y_pred)

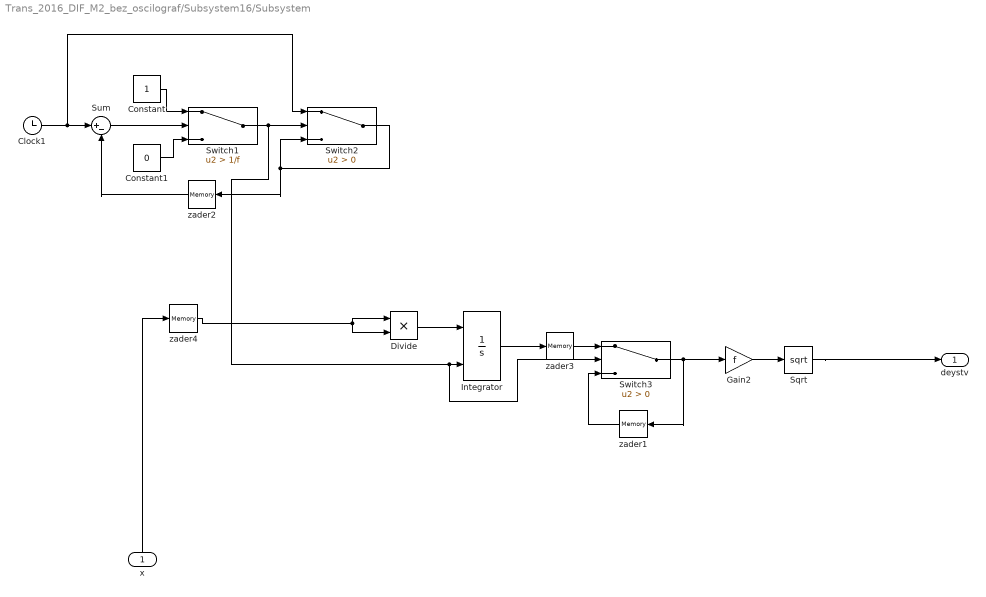
== system Trans_2016_DIF_M2_bez_oscilograf/Subsystem16/Subsystem ==
  x : Inport
  Clock1 : Clock
  Constant : Constant
  Constant1 : Constant  Value=0
  Divide : Product  Inputs=**
  Gain2 : Gain  Gain=f
  Integrator : Integrator  ExternalReset=level
  Sqrt : Sqrt  SaturateOnIntegerOverflow=on
  Sum : Sum  Inputs=|+-
  Switch1 : Switch  Criteria=u2 > Threshold  Threshold=1/f
  Switch2 : Switch  Criteria=u2 > Threshold
  Switch3 : Switch  Criteria=u2 > Threshold
  zader{1..4} (4 alike) : Memory
  deystv : Outport
  wires:
  zader4/1 -> Divide/2, Divide/1
  zader3/1 -> Switch3/1
  zader1/1 -> Switch3/3
  zader2/1 -> Sum/2
  Gain2/1 -> Sqrt/1
  Sqrt/1 -> deystv/1
  Switch3/1 -> zader1/1, Gain2/1
  Divide/1 -> Integrator/1
  Sum/1 -> Switch1/2
  Constant1/1 -> Switch1/3
  Switch1/1 -> Switch2/2, Integrator/2, Switch3/2
  Constant/1 -> Switch1/1
  x/1 -> zader4/1
  Switch2/1 -> Switch2/3, zader2/1
  Clock1/1 -> Sum/1, Switch2/1
  Integrator/1 -> zader3/1

== system Trans_2016_DIF_M2_bez_oscilograf/Subsystem16/Subsystem4 ==
  х : Inport
  Clock1 : Clock
  Constant : Constant  Value=T
  MATLAB Function : MATLAB Function  TreatAsAtomicUnit=on
  zader : Memory
  zader1 : Memory
  фаза : Outport
  wires:
  zader1/1 -> MATLAB Function/5(y_pred)
  Constant/1 -> MATLAB Function/2(T_period)
  х/1 -> MATLAB Function/3(x), zader/1
  Clock1/1 -> MATLAB Function/1(t)
  zader/1 -> MATLAB Function/4(x_pred)
  MATLAB Function/1(y) -> zader1/1, фаза/1

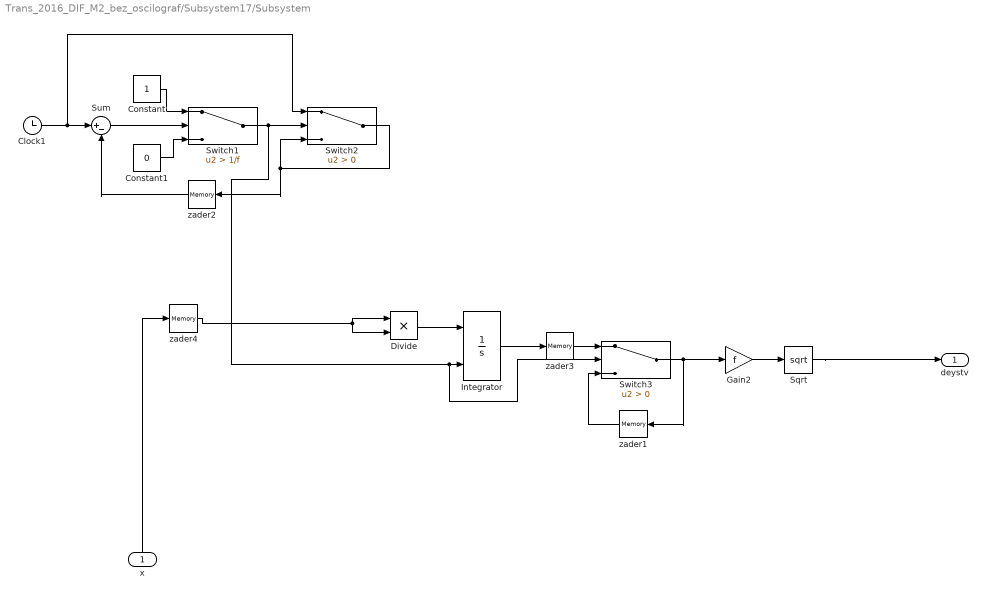
== system Trans_2016_DIF_M2_bez_oscilograf/Subsystem17/Subsystem ==
  x : Inport
  Clock1 : Clock
  Constant : Constant
  Constant1 : Constant  Value=0
  Divide : Product  Inputs=**
  Gain2 : Gain  Gain=f
  Integrator : Integrator  ExternalReset=level
  Sqrt : Sqrt  SaturateOnIntegerOverflow=on
  Sum : Sum  Inputs=|+-
  Switch1 : Switch  Criteria=u2 > Threshold  Threshold=1/f
  Switch2 : Switch  Criteria=u2 > Threshold
  Switch3 : Switch  Criteria=u2 > Threshold
  zader{1..4} (4 alike) : Memory
  deystv : Outport
  wires:
  Integrator/1 -> zader3/1
  Clock1/1 -> Switch2/1, Sum/1
  Switch2/1 -> zader2/1, Switch2/3
  x/1 -> zader4/1
  Constant/1 -> Switch1/1
  Switch1/1 -> Switch3/2, Integrator/2, Switch2/2
  Constant1/1 -> Switch1/3
  Sum/1 -> Switch1/2
  Divide/1 -> Integrator/1
  Switch3/1 -> Gain2/1, zader1/1
  Sqrt/1 -> deystv/1
  Gain2/1 -> Sqrt/1
  zader2/1 -> Sum/2
  zader1/1 -> Switch3/3
  zader3/1 -> Switch3/1
  zader4/1 -> Divide/1, Divide/2

== system Trans_2016_DIF_M2_bez_oscilograf/Subsystem17/Subsystem4 ==
  х : Inport
  Clock1 : Clock
  Constant : Constant  Value=T
  MATLAB Function : MATLAB Function  TreatAsAtomicUnit=on
  zader : Memory
  zader1 : Memory
  фаза : Outport
  wires:
  MATLAB Function/1(y) -> фаза/1, zader1/1
  zader/1 -> MATLAB Function/4(x_pred)
  Clock1/1 -> MATLAB Function/1(t)
  х/1 -> zader/1, MATLAB Function/3(x)
  Constant/1 -> MATLAB Function/2(T_period)
  zader1/1 -> MATLAB Function/5(y_pred)

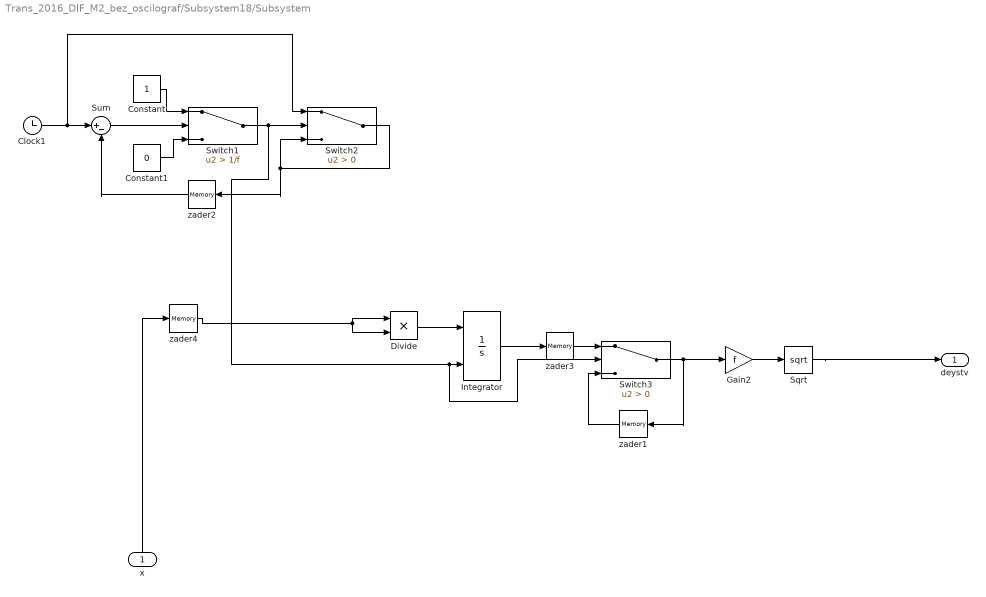
== system Trans_2016_DIF_M2_bez_oscilograf/Subsystem18/Subsystem ==
  x : Inport
  Clock1 : Clock
  Constant : Constant
  Constant1 : Constant  Value=0
  Divide : Product  Inputs=**
  Gain2 : Gain  Gain=f
  Integrator : Integrator  ExternalReset=level
  Sqrt : Sqrt  SaturateOnIntegerOverflow=on
  Sum : Sum  Inputs=|+-
  Switch1 : Switch  Criteria=u2 > Threshold  Threshold=1/f
  Switch2 : Switch  Criteria=u2 > Threshold
  Switch3 : Switch  Criteria=u2 > Threshold
  zader{1..4} (4 alike) : Memory
  deystv : Outport
  wires:
  zader4/1 -> Divide/2, Divide/1
  zader3/1 -> Switch3/1
  zader1/1 -> Switch3/3
  zader2/1 -> Sum/2
  Gain2/1 -> Sqrt/1
  Sqrt/1 -> deystv/1
  Switch3/1 -> zader1/1, Gain2/1
  Divide/1 -> Integrator/1
  Sum/1 -> Switch1/2
  Constant1/1 -> Switch1/3
  Switch1/1 -> Switch2/2, Integrator/2, Switch3/2
  Constant/1 -> Switch1/1
  x/1 -> zader4/1
  Switch2/1 -> Switch2/3, zader2/1
  Clock1/1 -> Sum/1, Switch2/1
  Integrator/1 -> zader3/1

== system Trans_2016_DIF_M2_bez_oscilograf/Subsystem18/Subsystem4 ==
  х : Inport
  Clock1 : Clock
  Constant : Constant  Value=T
  MATLAB Function : MATLAB Function  TreatAsAtomicUnit=on
  zader : Memory
  zader1 : Memory
  фаза : Outport
  wires:
  zader1/1 -> MATLAB Function/5(y_pred)
  Constant/1 -> MATLAB Function/2(T_period)
  х/1 -> MATLAB Function/3(x), zader/1
  Clock1/1 -> MATLAB Function/1(t)
  zader/1 -> MATLAB Function/4(x_pred)
  MATLAB Function/1(y) -> zader1/1, фаза/1

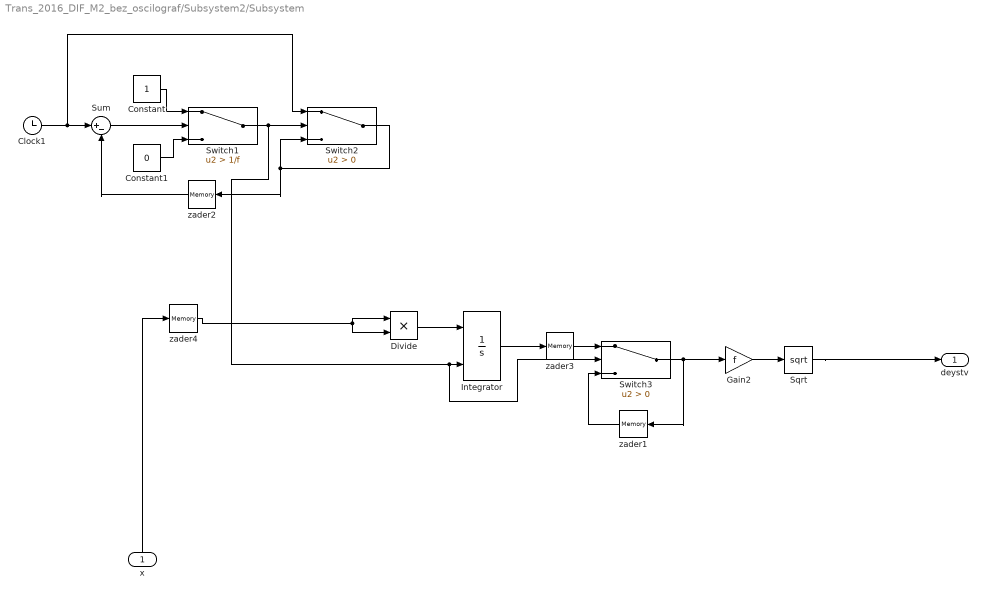
== system Trans_2016_DIF_M2_bez_oscilograf/Subsystem2/Subsystem ==
  x : Inport
  Clock1 : Clock
  Constant : Constant
  Constant1 : Constant  Value=0
  Divide : Product  Inputs=**
  Gain2 : Gain  Gain=f
  Integrator : Integrator  ExternalReset=level
  Sqrt : Sqrt  SaturateOnIntegerOverflow=on
  Sum : Sum  Inputs=|+-
  Switch1 : Switch  Criteria=u2 > Threshold  Threshold=1/f
  Switch2 : Switch  Criteria=u2 > Threshold
  Switch3 : Switch  Criteria=u2 > Threshold
  zader{1..4} (4 alike) : Memory
  deystv : Outport
  wires:
  zader4/1 -> Divide/2, Divide/1
  zader3/1 -> Switch3/1
  zader1/1 -> Switch3/3
  zader2/1 -> Sum/2
  Gain2/1 -> Sqrt/1
  Sqrt/1 -> deystv/1
  Switch3/1 -> zader1/1, Gain2/1
  Divide/1 -> Integrator/1
  Sum/1 -> Switch1/2
  Constant1/1 -> Switch1/3
  Switch1/1 -> Switch2/2, Integrator/2, Switch3/2
  Constant/1 -> Switch1/1
  x/1 -> zader4/1
  Switch2/1 -> Switch2/3, zader2/1
  Clock1/1 -> Sum/1, Switch2/1
  Integrator/1 -> zader3/1

== system Trans_2016_DIF_M2_bez_oscilograf/Subsystem2/Subsystem4 ==
  х : Inport
  Clock1 : Clock
  Constant : Constant  Value=T
  MATLAB Function : MATLAB Function  TreatAsAtomicUnit=on
  zader : Memory
  zader1 : Memory
  фаза : Outport
  wires:
  zader1/1 -> MATLAB Function/5(y_pred)
  Constant/1 -> MATLAB Function/2(T_period)
  х/1 -> MATLAB Function/3(x), zader/1
  Clock1/1 -> MATLAB Function/1(t)
  zader/1 -> MATLAB Function/4(x_pred)
  MATLAB Function/1(y) -> zader1/1, фаза/1

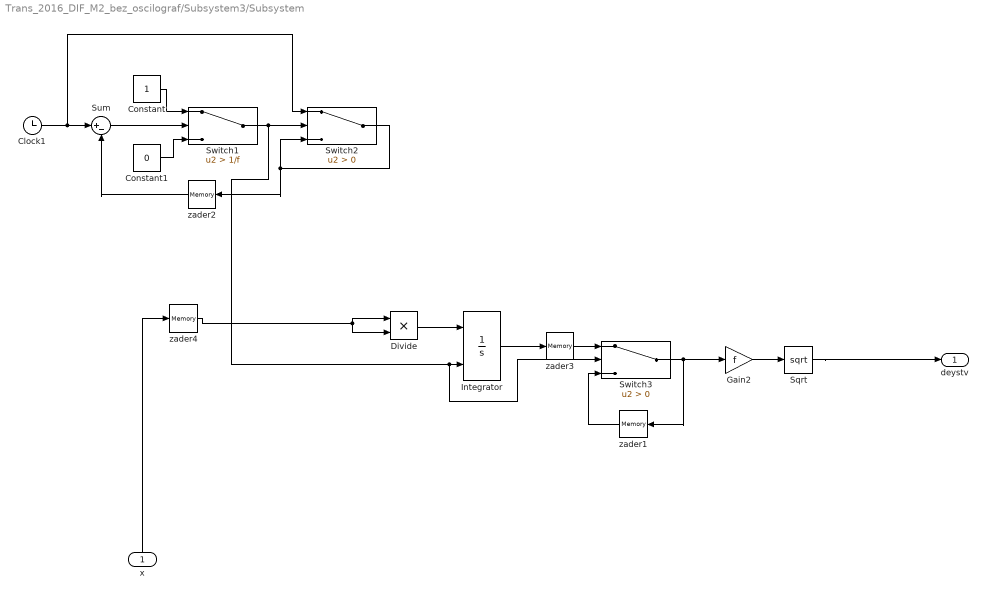
== system Trans_2016_DIF_M2_bez_oscilograf/Subsystem3/Subsystem ==
  x : Inport
  Clock1 : Clock
  Constant : Constant
  Constant1 : Constant  Value=0
  Divide : Product  Inputs=**
  Gain2 : Gain  Gain=f
  Integrator : Integrator  ExternalReset=level
  Sqrt : Sqrt  SaturateOnIntegerOverflow=on
  Sum : Sum  Inputs=|+-
  Switch1 : Switch  Criteria=u2 > Threshold  Threshold=1/f
  Switch2 : Switch  Criteria=u2 > Threshold
  Switch3 : Switch  Criteria=u2 > Threshold
  zader{1..4} (4 alike) : Memory
  deystv : Outport
  wires:
  Integrator/1 -> zader3/1
  Clock1/1 -> Switch2/1, Sum/1
  Switch2/1 -> zader2/1, Switch2/3
  x/1 -> zader4/1
  Constant/1 -> Switch1/1
  Switch1/1 -> Switch3/2, Integrator/2, Switch2/2
  Constant1/1 -> Switch1/3
  Sum/1 -> Switch1/2
  Divide/1 -> Integrator/1
  Switch3/1 -> Gain2/1, zader1/1
  Sqrt/1 -> deystv/1
  Gain2/1 -> Sqrt/1
  zader2/1 -> Sum/2
  zader1/1 -> Switch3/3
  zader3/1 -> Switch3/1
  zader4/1 -> Divide/1, Divide/2

== system Trans_2016_DIF_M2_bez_oscilograf/Subsystem3/Subsystem4 ==
  х : Inport
  Clock1 : Clock
  Constant : Constant  Value=T
  MATLAB Function : MATLAB Function  TreatAsAtomicUnit=on
  zader : Memory
  zader1 : Memory
  фаза : Outport
  wires:
  MATLAB Function/1(y) -> фаза/1, zader1/1
  zader/1 -> MATLAB Function/4(x_pred)
  Clock1/1 -> MATLAB Function/1(t)
  х/1 -> zader/1, MATLAB Function/3(x)
  Constant/1 -> MATLAB Function/2(T_period)
  zader1/1 -> MATLAB Function/5(y_pred)

== system Trans_2016_DIF_M2_bez_oscilograf/Subsystem4/Subsystem ==
  x : Inport
  Clock1 : Clock
  Constant : Constant
  Constant1 : Constant  Value=0
  Divide : Product  Inputs=**
  Gain2 : Gain  Gain=f
  Integrator : Integrator  ExternalReset=level
  Sqrt : Sqrt  SaturateOnIntegerOverflow=on
  Sum : Sum  Inputs=|+-
  Switch1 : Switch  Criteria=u2 > Threshold  Threshold=1/f
  Switch2 : Switch  Criteria=u2 > Threshold
  Switch3 : Switch  Criteria=u2 > Threshold
  zader{1..4} (4 alike) : Memory
  deystv : Outport
  wires:
  zader4/1 -> Divide/2, Divide/1
  zader3/1 -> Switch3/1
  zader1/1 -> Switch3/3
  zader2/1 -> Sum/2
  Gain2/1 -> Sqrt/1
  Sqrt/1 -> deystv/1
  Switch3/1 -> zader1/1, Gain2/1
  Divide/1 -> Integrator/1
  Sum/1 -> Switch1/2
  Constant1/1 -> Switch1/3
  Switch1/1 -> Switch2/2, Integrator/2, Switch3/2
  Constant/1 -> Switch1/1
  x/1 -> zader4/1
  Switch2/1 -> Switch2/3, zader2/1
  Clock1/1 -> Sum/1, Switch2/1
  Integrator/1 -> zader3/1

== system Trans_2016_DIF_M2_bez_oscilograf/Subsystem4/Subsystem4 ==
  х : Inport
  Clock1 : Clock
  Constant : Constant  Value=T
  MATLAB Function : MATLAB Function  TreatAsAtomicUnit=on
  zader : Memory
  zader1 : Memory
  фаза : Outport
  wires:
  zader1/1 -> MATLAB Function/5(y_pred)
  Constant/1 -> MATLAB Function/2(T_period)
  х/1 -> MATLAB Function/3(x), zader/1
  Clock1/1 -> MATLAB Function/1(t)
  zader/1 -> MATLAB Function/4(x_pred)
  MATLAB Function/1(y) -> zader1/1, фаза/1

== system Trans_2016_DIF_M2_bez_oscilograf/Subsystem5/Subsystem ==
  x : Inport
  Clock1 : Clock
  Constant : Constant
  Constant1 : Constant  Value=0
  Divide : Product  Inputs=**
  Gain2 : Gain  Gain=f
  Integrator : Integrator  ExternalReset=level
  Sqrt : Sqrt  SaturateOnIntegerOverflow=on
  Sum : Sum  Inputs=|+-
  Switch1 : Switch  Criteria=u2 > Threshold  Threshold=1/f
  Switch2 : Switch  Criteria=u2 > Threshold
  Switch3 : Switch  Criteria=u2 > Threshold
  zader{1..4} (4 alike) : Memory
  deystv : Outport
  wires:
  Integrator/1 -> zader3/1
  Clock1/1 -> Switch2/1, Sum/1
  Switch2/1 -> zader2/1, Switch2/3
  x/1 -> zader4/1
  Constant/1 -> Switch1/1
  Switch1/1 -> Switch3/2, Integrator/2, Switch2/2
  Constant1/1 -> Switch1/3
  Sum/1 -> Switch1/2
  Divide/1 -> Integrator/1
  Switch3/1 -> Gain2/1, zader1/1
  Sqrt/1 -> deystv/1
  Gain2/1 -> Sqrt/1
  zader2/1 -> Sum/2
  zader1/1 -> Switch3/3
  zader3/1 -> Switch3/1
  zader4/1 -> Divide/1, Divide/2

== system Trans_2016_DIF_M2_bez_oscilograf/Subsystem5/Subsystem4 ==
  х : Inport
  Clock1 : Clock
  Constant : Constant  Value=T
  MATLAB Function : MATLAB Function  TreatAsAtomicUnit=on
  zader : Memory
  zader1 : Memory
  фаза : Outport
  wires:
  MATLAB Function/1(y) -> фаза/1, zader1/1
  zader/1 -> MATLAB Function/4(x_pred)
  Clock1/1 -> MATLAB Function/1(t)
  х/1 -> zader/1, MATLAB Function/3(x)
  Constant/1 -> MATLAB Function/2(T_period)
  zader1/1 -> MATLAB Function/5(y_pred)

== system Trans_2016_DIF_M2_bez_oscilograf/Subsystem6/Subsystem ==
  x : Inport
  Clock1 : Clock
  Constant : Constant
  Constant1 : Constant  Value=0
  Divide : Product  Inputs=**
  Gain2 : Gain  Gain=f
  Integrator : Integrator  ExternalReset=level
  Sqrt : Sqrt  SaturateOnIntegerOverflow=on
  Sum : Sum  Inputs=|+-
  Switch1 : Switch  Criteria=u2 > Threshold  Threshold=1/f
  Switch2 : Switch  Criteria=u2 > Threshold
  Switch3 : Switch  Criteria=u2 > Threshold
  zader{1..4} (4 alike) : Memory
  deystv : Outport
  wires:
  zader4/1 -> Divide/2, Divide/1
  zader3/1 -> Switch3/1
  zader1/1 -> Switch3/3
  zader2/1 -> Sum/2
  Gain2/1 -> Sqrt/1
  Sqrt/1 -> deystv/1
  Switch3/1 -> zader1/1, Gain2/1
  Divide/1 -> Integrator/1
  Sum/1 -> Switch1/2
  Constant1/1 -> Switch1/3
  Switch1/1 -> Switch2/2, Integrator/2, Switch3/2
  Constant/1 -> Switch1/1
  x/1 -> zader4/1
  Switch2/1 -> Switch2/3, zader2/1
  Clock1/1 -> Sum/1, Switch2/1
  Integrator/1 -> zader3/1

== system Trans_2016_DIF_M2_bez_oscilograf/Subsystem6/Subsystem4 ==
  х : Inport
  Clock1 : Clock
  Constant : Constant  Value=T
  MATLAB Function : MATLAB Function  TreatAsAtomicUnit=on
  zader : Memory
  zader1 : Memory
  фаза : Outport
  wires:
  zader1/1 -> MATLAB Function/5(y_pred)
  Constant/1 -> MATLAB Function/2(T_period)
  х/1 -> MATLAB Function/3(x), zader/1
  Clock1/1 -> MATLAB Function/1(t)
  zader/1 -> MATLAB Function/4(x_pred)
  MATLAB Function/1(y) -> zader1/1, фаза/1

== system Trans_2016_DIF_M2_bez_oscilograf/Subsystem7/Subsystem ==
  x : Inport
  Clock1 : Clock
  Constant : Constant
  Constant1 : Constant  Value=0
  Divide : Product  Inputs=**
  Gain2 : Gain  Gain=f
  Integrator : Integrator  ExternalReset=level
  Sqrt : Sqrt  SaturateOnIntegerOverflow=on
  Sum : Sum  Inputs=|+-
  Switch1 : Switch  Criteria=u2 > Threshold  Threshold=1/f
  Switch2 : Switch  Criteria=u2 > Threshold
  Switch3 : Switch  Criteria=u2 > Threshold
  zader{1..4} (4 alike) : Memory
  deystv : Outport
  wires:
  Integrator/1 -> zader3/1
  Clock1/1 -> Switch2/1, Sum/1
  Switch2/1 -> zader2/1, Switch2/3
  x/1 -> zader4/1
  Constant/1 -> Switch1/1
  Switch1/1 -> Switch3/2, Integrator/2, Switch2/2
  Constant1/1 -> Switch1/3
  Sum/1 -> Switch1/2
  Divide/1 -> Integrator/1
  Switch3/1 -> Gain2/1, zader1/1
  Sqrt/1 -> deystv/1
  Gain2/1 -> Sqrt/1
  zader2/1 -> Sum/2
  zader1/1 -> Switch3/3
  zader3/1 -> Switch3/1
  zader4/1 -> Divide/1, Divide/2

== system Trans_2016_DIF_M2_bez_oscilograf/Subsystem7/Subsystem4 ==
  х : Inport
  Clock1 : Clock
  Constant : Constant  Value=T
  MATLAB Function : MATLAB Function  TreatAsAtomicUnit=on
  zader : Memory
  zader1 : Memory
  фаза : Outport
  wires:
  MATLAB Function/1(y) -> фаза/1, zader1/1
  zader/1 -> MATLAB Function/4(x_pred)
  Clock1/1 -> MATLAB Function/1(t)
  х/1 -> zader/1, MATLAB Function/3(x)
  Constant/1 -> MATLAB Function/2(T_period)
  zader1/1 -> MATLAB Function/5(y_pred)

== system Trans_2016_DIF_M2_bez_oscilograf/Subsystem8/Subsystem ==
  x : Inport
  Clock1 : Clock
  Constant : Constant
  Constant1 : Constant  Value=0
  Divide : Product  Inputs=**
  Gain2 : Gain  Gain=f
  Integrator : Integrator  ExternalReset=level
  Sqrt : Sqrt  SaturateOnIntegerOverflow=on
  Sum : Sum  Inputs=|+-
  Switch1 : Switch  Criteria=u2 > Threshold  Threshold=1/f
  Switch2 : Switch  Criteria=u2 > Threshold
  Switch3 : Switch  Criteria=u2 > Threshold
  zader{1..4} (4 alike) : Memory
  deystv : Outport
  wires:
  zader4/1 -> Divide/2, Divide/1
  zader3/1 -> Switch3/1
  zader1/1 -> Switch3/3
  zader2/1 -> Sum/2
  Gain2/1 -> Sqrt/1
  Sqrt/1 -> deystv/1
  Switch3/1 -> zader1/1, Gain2/1
  Divide/1 -> Integrator/1
  Sum/1 -> Switch1/2
  Constant1/1 -> Switch1/3
  Switch1/1 -> Switch2/2, Integrator/2, Switch3/2
  Constant/1 -> Switch1/1
  x/1 -> zader4/1
  Switch2/1 -> Switch2/3, zader2/1
  Clock1/1 -> Sum/1, Switch2/1
  Integrator/1 -> zader3/1

== system Trans_2016_DIF_M2_bez_oscilograf/Subsystem8/Subsystem4 ==
  х : Inport
  Clock1 : Clock
  Constant : Constant  Value=T
  MATLAB Function : MATLAB Function  TreatAsAtomicUnit=on
  zader : Memory
  zader1 : Memory
  фаза : Outport
  wires:
  zader1/1 -> MATLAB Function/5(y_pred)
  Constant/1 -> MATLAB Function/2(T_period)
  х/1 -> MATLAB Function/3(x), zader/1
  Clock1/1 -> MATLAB Function/1(t)
  zader/1 -> MATLAB Function/4(x_pred)
  MATLAB Function/1(y) -> zader1/1, фаза/1

== system Trans_2016_DIF_M2_bez_oscilograf/Subsystem9/Subsystem ==
  x : Inport
  Clock1 : Clock
  Constant : Constant
  Constant1 : Constant  Value=0
  Divide : Product  Inputs=**
  Gain2 : Gain  Gain=f
  Integrator : Integrator  ExternalReset=level
  Sqrt : Sqrt  SaturateOnIntegerOverflow=on
  Sum : Sum  Inputs=|+-
  Switch1 : Switch  Criteria=u2 > Threshold  Threshold=1/f
  Switch2 : Switch  Criteria=u2 > Threshold
  Switch3 : Switch  Criteria=u2 > Threshold
  zader{1..4} (4 alike) : Memory
  deystv : Outport
  wires:
  Integrator/1 -> zader3/1
  Clock1/1 -> Switch2/1, Sum/1
  Switch2/1 -> zader2/1, Switch2/3
  x/1 -> zader4/1
  Constant/1 -> Switch1/1
  Switch1/1 -> Switch3/2, Integrator/2, Switch2/2
  Constant1/1 -> Switch1/3
  Sum/1 -> Switch1/2
  Divide/1 -> Integrator/1
  Switch3/1 -> Gain2/1, zader1/1
  Sqrt/1 -> deystv/1
  Gain2/1 -> Sqrt/1
  zader2/1 -> Sum/2
  zader1/1 -> Switch3/3
  zader3/1 -> Switch3/1
  zader4/1 -> Divide/1, Divide/2

== system Trans_2016_DIF_M2_bez_oscilograf/Subsystem9/Subsystem4 ==
  х : Inport
  Clock1 : Clock
  Constant : Constant  Value=T
  MATLAB Function : MATLAB Function  TreatAsAtomicUnit=on
  zader : Memory
  zader1 : Memory
  фаза : Outport
  wires:
  MATLAB Function/1(y) -> фаза/1, zader1/1
  zader/1 -> MATLAB Function/4(x_pred)
  Clock1/1 -> MATLAB Function/1(t)
  х/1 -> zader/1, MATLAB Function/3(x)
  Constant/1 -> MATLAB Function/2(T_period)
  zader1/1 -> MATLAB Function/5(y_pred)

== system Trans_2016_DIF_M2_bez_oscilograf/модель трансформатора2/Form_Lsigma ==
  C : Inport
  Constant : Constant  Value=w1
  Constant1 : Constant  Value=w2
  Constant11 : Constant  Value=Lsigmavx
  MATLAB Function : MATLAB Function  TreatAsAtomicUnit=on
  Lsigma : Outport
  wires:
  Constant11/1 -> MATLAB Function/1(LsigmaX)
  C/1 -> MATLAB Function/2(C)
  MATLAB Function/1(Lsigma) -> Lsigma/1
  Constant/1 -> MATLAB Function/3(w1)
  Constant1/1 -> MATLAB Function/4(w2)

== system Trans_2016_DIF_M2_bez_oscilograf/модель трансформатора2/Ra1 ==
  Breaker1 : powerlib/Elements/Breaker  InitialState=0  SwitchingTimes="[t  1e6]"  External=off  BreakerResistance=1e-4  SnubberResistance=1e10  SnubberCapacitance=inf  Measurements=None  MoreParameters=on  NoBreakLoop=off
  Parallel RLC Branch : powerlib/Elements/Parallel RLC Branch  LConnTagsString=a  RConnTagsString=__new0  BranchType=R  Resistance=r  Inductance=1e-3  SetiL0=off  InitialCurrent=0  Capacitance=1e-6  Setx0=off  InitialVoltage=0  Measurements=None
  "  " : PMIOPort  Port=1  Side=Right
  " " : PMIOPort  Port=2  Side=Left
  connections:
  " "/RConn1 -- Breaker1/LConn1
  Parallel RLC Branch/LConn1 -- Breaker1/RConn1
  "  "/RConn1 -- Parallel RLC Branch/RConn1

== system Trans_2016_DIF_M2_bez_oscilograf/модель трансформатора2/Rb1 ==
  Breaker1 : powerlib/Elements/Breaker  InitialState=0  SwitchingTimes="[t  1e6]"  External=off  BreakerResistance=1e-4  SnubberResistance=1e10  SnubberCapacitance=inf  Measurements=None  MoreParameters=on  NoBreakLoop=off
  Parallel RLC Branch : powerlib/Elements/Parallel RLC Branch  LConnTagsString=a  RConnTagsString=__new0  BranchType=R  Resistance=r  Inductance=1e-3  SetiL0=off  InitialCurrent=0  Capacitance=1e-6  Setx0=off  InitialVoltage=0  Measurements=None
  "  " : PMIOPort  Port=1  Side=Right
  " " : PMIOPort  Port=2  Side=Left
  connections:
  "  "/RConn1 -- Parallel RLC Branch/RConn1
  Parallel RLC Branch/LConn1 -- Breaker1/RConn1
  " "/RConn1 -- Breaker1/LConn1

== system Trans_2016_DIF_M2_bez_oscilograf/модель трансформатора2/Rc1 ==
  Breaker1 : powerlib/Elements/Breaker  InitialState=0  SwitchingTimes="[t  1e6]"  External=off  BreakerResistance=1e-4  SnubberResistance=1e10  SnubberCapacitance=inf  Measurements=None  MoreParameters=on  NoBreakLoop=off
  Parallel RLC Branch : powerlib/Elements/Parallel RLC Branch  LConnTagsString=a  RConnTagsString=__new0  BranchType=R  Resistance=r  Inductance=1e-3  SetiL0=off  InitialCurrent=0  Capacitance=1e-6  Setx0=off  InitialVoltage=0  Measurements=None
  "  " : PMIOPort  Port=1  Side=Right
  " " : PMIOPort  Port=2  Side=Left
  connections:
  " "/RConn1 -- Breaker1/LConn1
  Parallel RLC Branch/LConn1 -- Breaker1/RConn1
  "  "/RConn1 -- Parallel RLC Branch/RConn1
